simulink model "kiteModelNoAddedMassRapp"  (R2022a)
settings: Solver=VariableStepAuto  StartTime=0.0  StopTime=10.0  RelTol=1e-3
values from neighbouring files (symbols this model uses):
  aileronCmd = 0    [kiteModelNoAddedMassRapp_ts.m]
  alphaaI = 5    [kiteModelNoAddedMassRapp_ts.m]
  azI = 0    [kiteModelNoAddedMassRapp_ts.m]
  betaaI = 5    [kiteModelNoAddedMassRapp_ts.m]
  elevatorCmd = 4    [kiteModelNoAddedMassRapp_ts.m]
  elI = 20    [kiteModelNoAddedMassRapp_ts.m]
  htI = 100    [kiteModelNoAddedMassRapp_ts.m]
  J = vhcl.inertia_CM.Value    [kiteModelNoAddedMassRapp_ts.m]
  Jinv = inv(J)    [kiteModelNoAddedMassRapp_ts.m]
  m = vhcl.mass.Value    [kiteModelNoAddedMassRapp_ts.m]
  pbI = 0    [kiteModelNoAddedMassRapp_ts.m]
  phitI = 0    [kiteModelNoAddedMassRapp_ts.m]
  psitI = 0    [kiteModelNoAddedMassRapp_ts.m]
  qbI = 0    [kiteModelNoAddedMassRapp_ts.m]
  rbI = 0    [kiteModelNoAddedMassRapp_ts.m]
  rudderCmd = 0    [kiteModelNoAddedMassRapp_ts.m]
  thetatI = 0    [kiteModelNoAddedMassRapp_ts.m]
  vaI = 5    [kiteModelNoAddedMassRapp_ts.m]
  vW = 1    [kiteModelNoAddedMassRapp_ts.m]
undefined symbols (not defined in the file or in its folder): Copy_of_fluidDynamicSurface_cl, fluidDynamicSurface, fThrTanZConstant, vhcl
libraries: vrlib x12, dynamicPressure_ul x4, Copy_of_clAndCdCalculator_cl x4, alphaBetaLE_ul x4, localApparentWind_ul x4, rotateAboutVec x4, matrix_library x1
settings Model: Creator=jcreed2  LastModifiedBy=jcreed2
settings DebuggingCC: AlgebraicLoopMsg=none  ArtificialAlgebraicLoopMsg=none

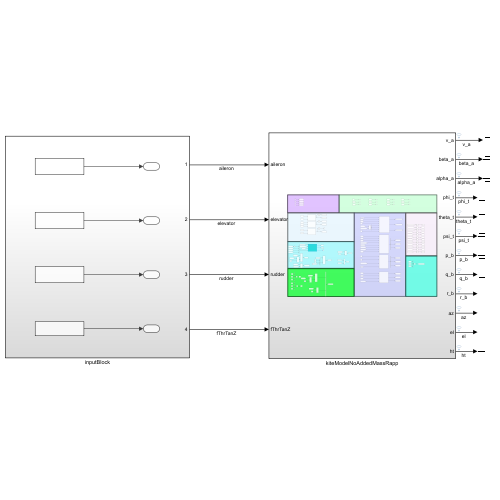
[thumbnail: Simulink's stored preview of the top-level diagram]
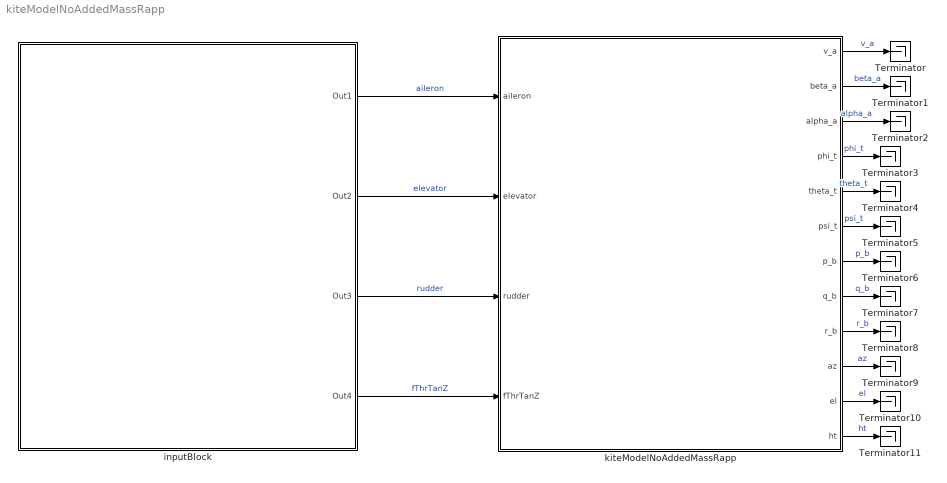
== system kiteModelNoAddedMassRapp ==
  Terminator{,1..11} (12 alike) : Terminator
  inputBlock : Subsystem
  kiteModelNoAddedMassRapp : Subsystem
  wires:
  kiteModelNoAddedMassRapp/1(v_a) -> Terminator/1  "v_a"
  kiteModelNoAddedMassRapp/2(beta_a) -> Terminator1/1  "beta_a"
  kiteModelNoAddedMassRapp/3(alpha_a) -> Terminator2/1  "alpha_a"
  kiteModelNoAddedMassRapp/4(phi_t) -> Terminator3/1  "phi_t"
  kiteModelNoAddedMassRapp/5(theta_t) -> Terminator4/1  "theta_t"
  kiteModelNoAddedMassRapp/6(psi_t) -> Terminator5/1  "psi_t"
  kiteModelNoAddedMassRapp/7(p_b) -> Terminator6/1  "p_b"
  kiteModelNoAddedMassRapp/8(q_b) -> Terminator7/1  "q_b"
  kiteModelNoAddedMassRapp/9(r_b) -> Terminator8/1  "r_b"
  kiteModelNoAddedMassRapp/10(az) -> Terminator9/1  "az"
  kiteModelNoAddedMassRapp/11(el) -> Terminator10/1  "el"
  kiteModelNoAddedMassRapp/12(ht) -> Terminator11/1  "ht"
  inputBlock/1(Out1) -> kiteModelNoAddedMassRapp/1(aileron)  "aileron"
  inputBlock/2(Out2) -> kiteModelNoAddedMassRapp/2(elevator)  "elevator"
  inputBlock/3(Out3) -> kiteModelNoAddedMassRapp/3(rudder)  "rudder"
  inputBlock/4(Out4) -> kiteModelNoAddedMassRapp/4(fThrTanZ)  "fThrTanZ"

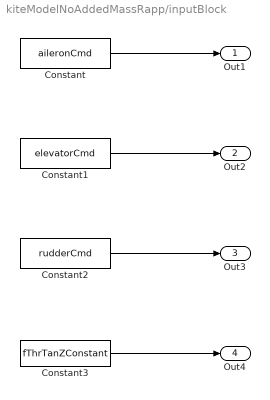
== system kiteModelNoAddedMassRapp/inputBlock ==
  Constant : Constant  Value=aileronCmd
  Constant1 : Constant  Value=elevatorCmd
  Constant2 : Constant  Value=rudderCmd
  Constant3 : Constant  Value=fThrTanZConstant
  Out1 : Outport
  Out2 : Outport  Port=2
  Out3 : Outport  Port=3
  Out4 : Outport  Port=4
  wires:
  Constant3/1 -> Out4/1
  Constant2/1 -> Out3/1
  Constant1/1 -> Out2/1
  Constant/1 -> Out1/1

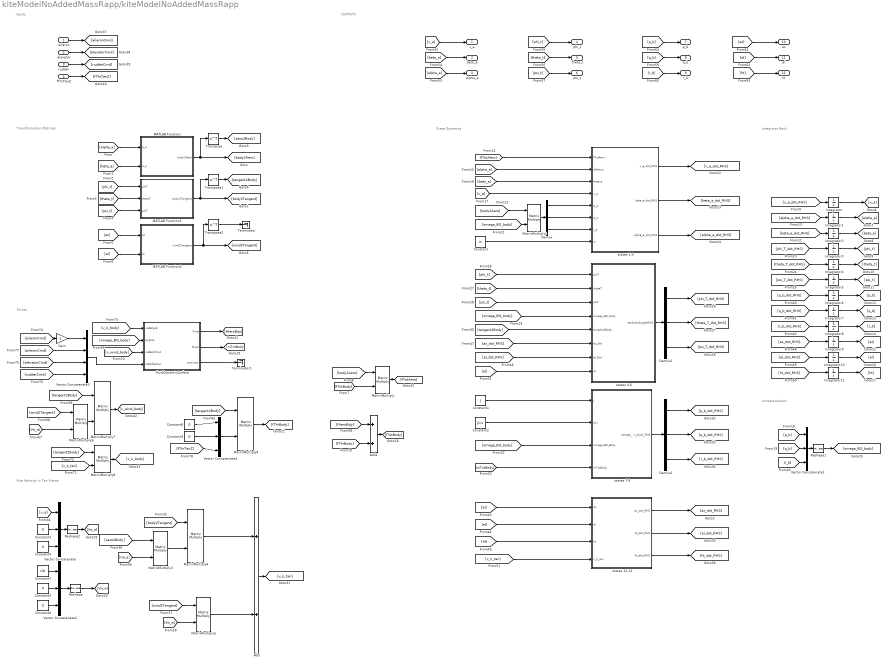
== system kiteModelNoAddedMassRapp/kiteModelNoAddedMassRapp ==
  note: OUTPUTS
  note: Inputs
  note: Kite Velocity in Tan Frame
  note: concatenations
  note: State Dynamics
  note: Forces
  note: Integrator Bank
  note: Transformation Matrices
  aileron : Inport
  elevator : Inport  Port=2
  rudder : Inport  Port=3
  fThrTanZ : Inport  Port=4
  Add : Sum
  Add1 : Sum
  Constant : Constant  Value=m
  Constant1 : Constant  Value=J
  Constant2 : Constant  Value=Jinv
  Constant{3..6,8..9} (6 alike) : Constant  Value=0
  Constant7 : Constant  Value=vW
  Demux : Demux  Outputs=3
  Demux1 : Demux  Outputs=3
  Demux2 : Demux  Outputs=3
  Gain : Gain  Gain=-1
  Integrator : Integrator  InitialCondition=vaI
  Integrator1 : Integrator  InitialCondition=alphaaI
  Integrator10 : Integrator  InitialCondition=elI
  Integrator11 : Integrator  InitialCondition=htI
  Integrator2 : Integrator  InitialCondition=betaaI
  Integrator3 : Integrator  InitialCondition=phitI
  Integrator4 : Integrator  InitialCondition=thetatI
  Integrator5 : Integrator  InitialCondition=psitI
  Integrator6 : Integrator  InitialCondition=pbI
  Integrator7 : Integrator  InitialCondition=qbI
  Integrator8 : Integrator  InitialCondition=rbI
  Integrator9 : Integrator  InitialCondition=azI
  MATLAB Function : MATLAB Function  TreatAsAtomicUnit=on
  MATLAB Function1 : MATLAB Function  TreatAsAtomicUnit=on
  MATLAB Function2 : MATLAB Function  TreatAsAtomicUnit=on
  MatrixMultiply{,2..9} (9 alike) : Product  Multiplication=Matrix(*)
  Reshape : Reshape  OutputDimensionality=Column vector (2-D)
  Reshape1 : Reshape  OutputDimensionality=Column vector (2-D)
  Reshape2 : Reshape  OutputDimensionality=Column vector (2-D)
  Terminator : Terminator
  Terminator1 : Terminator
  Transpose : Math  Operator=transpose
  Transpose1 : Math  Operator=transpose
  Transpose2 : Math  Operator=transpose
  Vector Concatenate{,1..2,4} (4 alike) : Concatenate  NumInputs=3
  Vector Concatenate3 : Concatenate  NumInputs=4
  fluidDynamicSurface : Subsystem  AncestorBlock=Copy_of_fluidDynamicSurface_cl/fluidDynamicSurface  mask{vcl=vhcl, fluidDensity=1000, fluidMomentArms=vhcl.fluidMomentArms.Value, fluidRefArea=vhcl.fluidRefArea.Value, wingTips=vhcl.wingTipPositions.Value}
      mask prompts: vcl "Vehicle object"; fluidDensity "Fluid density"; fluidMomentArms "Fluid Moment Arms"; fluidRefArea "Fluid Reference Area"; wingTips "Wing Tips"
      mask help:
      | Input must be an 1×N struct array with fields:
      |     refArea
      |     aeroCentPosVec
      |     spanUnitVec
      |     chordUnitVec
      |     CL
      |     CD
      |     alpha
      |     GainCL
      |     GainCD
      |
      | where N is the number of aerodynamic surfaces
      settings: MinAlgLoopOccurrences=on
  states 1-3 : Subsystem
  states 10-12 : Subsystem
  states 4-6 : Subsystem
  states 7-9 : Subsystem
  v_a : Outport
  beta_a : Outport  Port=2
  alpha_a : Outport  Port=3
  phi_t : Outport  Port=4
  theta_t : Outport  Port=5
  psi_t : Outport  Port=6
  p_b : Outport  Port=7
  q_b : Outport  Port=8
  r_b : Outport  Port=9
  az : Outport  Port=10
  el : Outport  Port=11
  ht : Outport  Port=12
  wires:
  Constant1/1 -> states 7-9/1(J)
  Constant2/1 -> states 7-9/2(Jinv)
  Demux/3 -> states 1-3/7(r_a)
  [omega_BO_body] -> states 7-9/3(omega_BO_Body)
  MatrixMultiply5/1 -> Add/2
  [tangent2Body] -> states 4-6/5(tangent2Body)
  [body2Aero] -> MatrixMultiply/1
  Integrator3/1 -> [phi_t]
  [phi_T_dot_RHS] -> Integrator3/1
  [body2Aero] -> MatrixMultiply2/1
  Integrator/1 -> [v_a]
  [el] -> states 4-6/8(el)
  Demux1/3 -> [psi_T_dot_RHS]
  states 1-3/2(beta_a_dot_RHS) -> [beta_a_dot_RHS]
  Constant6/1 -> Vector Concatenate2/3
  [psi_t] -> MATLAB Function1/3(psiT)
  Integrator1/1 -> [alpha_a]
  Vector Concatenate2/1 -> Reshape/1
  Transpose1/1 -> [tangent2Body]
  [Vw_w] -> MatrixMultiply5/2
  states 1-3/3(alpha_a_dot_RHS) -> [alpha_a_dot_RHS]
  Integrator5/1 -> [psi_t]
  [v_a] -> states 1-3/4(v_a)
  Integrator8/1 -> [r_b]
  Transpose/1 -> [aero2Body]
  Integrator4/1 -> [theta_t]
  [alpha_a] -> MATLAB Function/1(a_a)
  [alpha_a_dot_RHS] -> Integrator1/1
  [omega_BO_body] -> MatrixMultiply2/2
  states 10-12/3(ht_dot_RHS) -> [ht_dot_RHS]
  [r_b] -> Vector Concatenate1/3
  MatrixMultiply4/1 -> Add/1
  [theta_T_dot_RHS] -> Integrator4/1
  Integrator11/1 -> [ht]
  Demux/1 -> states 1-3/5(p_a)
  [beta_a_dot_RHS] -> Integrator2/1
  [p_b_dot_RHS] -> Integrator6/1
  [beta_a] -> MATLAB Function/2(b_a)
  Constant5/1 -> Vector Concatenate2/2
  [az] -> states 10-12/1(az)
  MATLAB Function/1(body2Aero) -> Transpose/1, [body2Aero]
  [v_a] -> Vector Concatenate/1
  Integrator6/1 -> [p_b]
  [v_k_tan] -> states 10-12/4(v_k_tan)
  [q_b_dot_RHS] -> Integrator7/1
  [phi_t] -> states 4-6/1(phiT)
  MatrixMultiply/1 -> [fTotAero]
  Integrator2/1 -> [beta_a]
  MatrixMultiply2/1 -> Demux/1
  Demux2/3 -> [r_b_dot_RHS]
  Integrator7/1 -> [q_b]
  states 7-9/1(omega_BO_Dot_body_RHS) -> Demux2/1
  Integrator10/1 -> [el]
  Reshape1/1 -> [omega_BO_body]
  [fTotBody] -> MatrixMultiply/2
  [el] -> MATLAB Function2/2(el)
  Constant3/1 -> Vector Concatenate/2
  MATLAB Function1/1(body2Tangent) -> Transpose1/1, [body2Tangent]
  [psi_t] -> states 4-6/3(psiT)
  MATLAB Function2/1(wind2Tangent) -> Transpose2/1, [wind2Tangent]
  [p_b] -> Vector Concatenate1/1
  [phi_t] -> MATLAB Function1/1(phiT)
  [q_b] -> Vector Concatenate1/2
  Integrator9/1 -> [az]
  [az_dot_RHS] -> Integrator9/1
  [ht_dot_RHS] -> Integrator11/1
  [az] -> MATLAB Function2/1(az)
  [theta_t] -> MATLAB Function1/2(thetaT)
  [r_b_dot_RHS] -> Integrator8/1
  [el_dot_RHS] -> Integrator10/1
  [mTotBody] -> states 7-9/4(mTotBody)
  [theta_t] -> states 4-6/2(thetaT)
  Constant7/1 -> Vector Concatenate2/1
  Demux/2 -> states 1-3/6(q_a)
  Vector Concatenate/1 -> Reshape2/1
  Transpose2/1 -> Terminator/1
  [fTotAero] -> states 1-3/1(fTotAero)
  [beta_a] -> states 1-3/3(beta_a)
  Demux1/2 -> [theta_T_dot_RHS]
  Demux1/1 -> [phi_T_dot_RHS]
  [body2Tangent] -> MatrixMultiply4/1
  [alpha_a] -> states 1-3/2(alpha_a)
  Demux2/2 -> [q_b_dot_RHS]
  [aero2Body] -> MatrixMultiply3/1
  [el_dot_RHS] -> states 4-6/7(el_Dot)
  Constant4/1 -> Vector Concatenate/3
  [psi_T_dot_RHS] -> Integrator5/1
  Constant/1 -> states 1-3/8(m)
  [el] -> states 10-12/2(el)
  [v_a_dot_RHS] -> Integrator/1
  states 1-3/1(v_a_dot_RHS) -> [v_a_dot_RHS]
  [ht] -> states 10-12/3(ht)
  MatrixMultiply3/1 -> MatrixMultiply4/2
  Demux2/1 -> [p_b_dot_RHS]
  states 10-12/1(az_dot_RHS) -> [az_dot_RHS]
  Vector Concatenate1/1 -> Reshape1/1
  states 10-12/2(el_dot_RHS) -> [el_dot_RHS]
  [Va_a] -> MatrixMultiply3/2
  Add/1 -> [v_k_tan]
  states 4-6/1(tanEulerAnglesRHS) -> Demux1/1
  [omega_BO_body] -> states 4-6/4(omega_BO_body)
  [wind2Tangent] -> MatrixMultiply5/1
  [az_dot_RHS] -> states 4-6/6(az_dot)
  Add1/1 -> [fTotBody]
  aileron/1 -> [aileronCmd]
  elevator/1 -> [elevatorCmd]
  rudder/1 -> [rudderCmd]
  fThrTanZ/1 -> [fThrTanZ]
  [alpha_a] -> alpha_a/1
  [beta_a] -> beta_a/1
  [v_a] -> v_a/1
  [phi_t] -> phi_t/1
  [theta_t] -> theta_t/1
  [psi_t] -> psi_t/1
  [p_b] -> p_b/1
  [q_b] -> q_b/1
  [r_b] -> r_b/1
  [az] -> az/1
  [el] -> el/1
  [ht] -> ht/1
  fluidDynamicSurface/3(powLoss) -> Terminator1/1
  fluidDynamicSurface/2(Mnet) -> [mTotBody]
  fluidDynamicSurface/1(Fnet) -> [fAeroBdy]
  [fAeroBdy] -> Add1/1
  [fThrBody] -> Add1/2
  [omega_BO_body] -> fluidDynamicSurface/2(angVel)
  [Vw_w] -> MatrixMultiply6/2
  [wind2Tangent] -> MatrixMultiply6/1
  MatrixMultiply6/1 -> MatrixMultiply7/2
  [tangent2Body] -> MatrixMultiply7/1
  MatrixMultiply7/1 -> [v_wind_body]
  [v_wind_body] -> fluidDynamicSurface/3(velBdyWind)
  [tangent2Body] -> MatrixMultiply8/1
  [v_k_tan] -> MatrixMultiply8/2
  MatrixMultiply8/1 -> [v_k_body]
  [v_k_body] -> fluidDynamicSurface/1(velBdyLE)
  Vector Concatenate3/1 -> fluidDynamicSurface/4(csDeflection)
  Gain/1 -> Vector Concatenate3/1
  [aileronCmd] -> Gain/1
  [elevatorCmd] -> Vector Concatenate3/3
  [rudderCmd] -> Vector Concatenate3/4
  [aileronCmd] -> Vector Concatenate3/2
  Reshape/1 -> [Vw_w]
  Reshape2/1 -> [Va_a]
  [fThrTanZ] -> Vector Concatenate4/3
  MatrixMultiply9/1 -> [fThrBody]
  [tangent2Body] -> MatrixMultiply9/1
  Vector Concatenate4/1 -> MatrixMultiply9/2
  Constant8/1 -> Vector Concatenate4/1
  Constant9/1 -> Vector Concatenate4/2

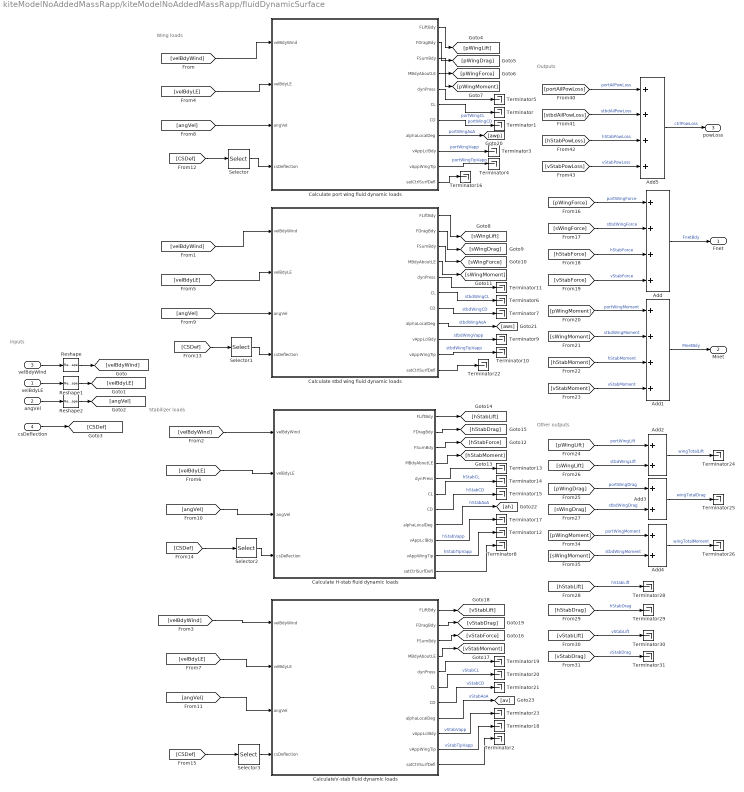
== system kiteModelNoAddedMassRapp/kiteModelNoAddedMassRapp/fluidDynamicSurface ==
  note: inputs
  note: Stabilizer loads
  note: WIng loads
  note: Outputs
  note: Other outputs
  velBdyLE : Inport
  angVel : Inport  Port=2
  velBdyWind : Inport  Port=3
  csDeflection : Inport  Port=4
  Add : Sum  Inputs=++++
  Add1 : Sum  Inputs=++++
  Add2 : Sum
  Add3 : Sum
  Add4 : Sum
  Add5 : Sum  Inputs=++++
  Calculate H-stab fluid dynamic loads : Subsystem  AncestorBlock=calcFluidDynamicLoads/Calculate fluid dynamic loads  mask{aSurf=vhcl.hStab, sRef=fluidRefArea, rArm_LE=fluidMomentArms(:,3), rTip_LE=wingTips(:,3), fluidDensity=fluidDensity}
      mask prompts: aSurf "Aerosurf object"; sRef "Reference area"; rArm_LE "Moment arm wrt wing LE"; rTip_LE "Surface tip wrt wing LE"; fluidDensity "Fluid density"
  Calculate port wing fluid dynamic loads : Subsystem  AncestorBlock=calcFluidDynamicLoads/Calculate fluid dynamic loads  mask{aSurf=vhcl.portWing, sRef=fluidRefArea, rArm_LE=fluidMomentArms(:,1), rTip_LE=wingTips(:,1), fluidDensity=fluidDensity}
      mask prompts: aSurf "Aerosurf object"; sRef "Reference area"; rArm_LE "Moment arm wrt wing LE"; rTip_LE "Surface tip wrt wing LE"; fluidDensity "Fluid density"
  Calculate stbd wing fluid dynamic loads : Subsystem  AncestorBlock=calcFluidDynamicLoads/Calculate fluid dynamic loads  mask{aSurf=vhcl.stbdWing, sRef=fluidRefArea, rArm_LE=fluidMomentArms(:,2), rTip_LE=wingTips(:,2), fluidDensity=fluidDensity}
      mask prompts: aSurf "Aerosurf object"; sRef "Reference area"; rArm_LE "Moment arm wrt wing LE"; rTip_LE "Surface tip wrt wing LE"; fluidDensity "Fluid density"
  CalculateV-stab fluid dynamic loads : Subsystem  AncestorBlock=calcFluidDynamicLoads/Calculate fluid dynamic loads  mask{aSurf=vhcl.vStab, sRef=fluidRefArea, rArm_LE=fluidMomentArms(:,4), rTip_LE=wingTips(:,4), fluidDensity=fluidDensity}
      mask prompts: aSurf "Aerosurf object"; sRef "Reference area"; rArm_LE "Moment arm wrt wing LE"; rTip_LE "Surface tip wrt wing LE"; fluidDensity "Fluid density"
  Reshape : Reshape  OutputDimensionality=Column vector (2-D)
  Reshape1 : Reshape  OutputDimensionality=Column vector (2-D)
  Reshape2 : Reshape  OutputDimensionality=Column vector (2-D)
  Selector : Selector  InputPortWidth=4  IndexOptions=Index vector (dialog)  Indices=1  OutputSizes=1
  Selector1 : Selector  InputPortWidth=4  IndexOptions=Index vector (dialog)  Indices=2  OutputSizes=1
  Selector2 : Selector  InputPortWidth=4  IndexOptions=Index vector (dialog)  Indices=3  OutputSizes=1
  Selector3 : Selector  InputPortWidth=4  IndexOptions=Index vector (dialog)  Indices=4  OutputSizes=1
  Terminator{,1..26,28..31} (31 alike) : Terminator
  Fnet : Outport
  Mnet : Outport  Port=2
  powLoss : Outport  Port=3
  wires:
  [vStabPowLoss] -> Add5/4  "vStabPowLoss"
  [hStabPowLoss] -> Add5/3  "hStabPowLoss"
  Add5/1 -> powLoss/1  "ctrlPowLoss"
  [stbdAilPowLoss] -> Add5/2  "stbdAilPowLoss"
  [portAilPowLoss] -> Add5/1  "portAilPowLoss"
  CalculateV-stab fluid dynamic loads/11(satCtrlSurfDefl) -> Terminator2/1
  Calculate H-stab fluid dynamic loads/11(satCtrlSurfDefl) -> Terminator8/1
  Calculate stbd wing fluid dynamic loads/11(satCtrlSurfDefl) -> Terminator22/1
  Calculate port wing fluid dynamic loads/11(satCtrlSurfDefl) -> Terminator16/1
  [sWingMoment] -> Add4/2  "stbdWingMoment"
  [pWingMoment] -> Add4/1  "portWingMoment"
  Add4/1 -> Terminator26/1  "wingTotalMoment"
  Add3/1 -> Terminator25/1  "wingTotalDrag"
  Add2/1 -> Terminator24/1  "wingTotalLift"
  [velBdyWind] -> CalculateV-stab fluid dynamic loads/1(velBdyWind)
  [velBdyWind] -> Calculate H-stab fluid dynamic loads/1(velBdyWind)
  [velBdyWind] -> Calculate stbd wing fluid dynamic loads/1(velBdyWind)
  [velBdyWind] -> Calculate port wing fluid dynamic loads/1(velBdyWind)
  [pWingLift] -> Add2/1  "portWingLift"
  [pWingDrag] -> Add3/1  "portWingDrag"
  [sWingLift] -> Add2/2  "stbdWingLift"
  [sWingDrag] -> Add3/2  "stbdWingDrag"
  [hStabLift] -> Terminator28/1  "hStabLift"
  [hStabDrag] -> Terminator29/1  "hStabDrag"
  [vStabLift] -> Terminator30/1  "vStabLift"
  [vStabDrag] -> Terminator31/1  "vStabDrag"
  [pWingMoment] -> Add1/1  "portWingMoment"
  [sWingMoment] -> Add1/2  "stbdWingMoment"
  [hStabMoment] -> Add1/3  "hStabMoment"
  [vStabMoment] -> Add1/4  "vStabMoment"
  Add1/1 -> Mnet/1  "MnetBdy"
  Add/1 -> Fnet/1  "FnetBdy"
  [hStabForce] -> Add/3  "hStabForce"
  [vStabForce] -> Add/4  "vStabForce"
  [sWingForce] -> Add/2  "stbdWingForce"
  [pWingForce] -> Add/1  "portWingForce"
  CalculateV-stab fluid dynamic loads/7(CD) -> Terminator21/1  "vStabCD"
  CalculateV-stab fluid dynamic loads/10(vAppWingTip) -> Terminator18/1  "vStabTipVapp"
  CalculateV-stab fluid dynamic loads/2(FDragBdy) -> [vStabDrag]
  CalculateV-stab fluid dynamic loads/5(dynPress) -> Terminator19/1
  CalculateV-stab fluid dynamic loads/8(alphaLocalDeg) -> [av]  "vStabAoA"
  CalculateV-stab fluid dynamic loads/4(MBdyAboutLE) -> [vStabMoment]
  CalculateV-stab fluid dynamic loads/9(vAppLclBdy) -> Terminator23/1  "vStabVapp"
  CalculateV-stab fluid dynamic loads/6(CL) -> Terminator20/1  "vStabCL"
  CalculateV-stab fluid dynamic loads/1(FLiftBdy) -> [vStabLift]
  CalculateV-stab fluid dynamic loads/3(FSumBdy) -> [vStabForce]
  Calculate H-stab fluid dynamic loads/9(vAppLclBdy) -> Terminator17/1  "hStabVapp"
  Calculate H-stab fluid dynamic loads/10(vAppWingTip) -> Terminator12/1  "hStabTipVapp"
  Calculate H-stab fluid dynamic loads/8(alphaLocalDeg) -> [ah]  "hStabAoA"
  Calculate H-stab fluid dynamic loads/3(FSumBdy) -> [hStabForce]
  Calculate H-stab fluid dynamic loads/6(CL) -> Terminator14/1  "hStabCL"
  Calculate H-stab fluid dynamic loads/1(FLiftBdy) -> [hStabLift]
  Calculate H-stab fluid dynamic loads/7(CD) -> Terminator15/1  "hStabCD"
  Calculate H-stab fluid dynamic loads/5(dynPress) -> Terminator13/1
  Calculate H-stab fluid dynamic loads/4(MBdyAboutLE) -> [hStabMoment]
  Calculate H-stab fluid dynamic loads/2(FDragBdy) -> [hStabDrag]
  Calculate stbd wing fluid dynamic loads/4(MBdyAboutLE) -> [sWingMoment]
  Calculate stbd wing fluid dynamic loads/3(FSumBdy) -> [sWingForce]
  Calculate stbd wing fluid dynamic loads/2(FDragBdy) -> [sWingDrag]
  Calculate stbd wing fluid dynamic loads/1(FLiftBdy) -> [sWingLift]
  Calculate stbd wing fluid dynamic loads/10(vAppWingTip) -> Terminator10/1  "stbdWingTipVapp"
  Calculate stbd wing fluid dynamic loads/7(CD) -> Terminator7/1  "stbdWingCD"
  Calculate stbd wing fluid dynamic loads/8(alphaLocalDeg) -> [aws]  "stbdWingAoA"
  Calculate stbd wing fluid dynamic loads/6(CL) -> Terminator6/1  "stbdWingCL"
  Calculate stbd wing fluid dynamic loads/9(vAppLclBdy) -> Terminator9/1  "stbdWingVapp"
  Calculate stbd wing fluid dynamic loads/5(dynPress) -> Terminator11/1
  Calculate port wing fluid dynamic loads/5(dynPress) -> Terminator5/1
  Calculate port wing fluid dynamic loads/10(vAppWingTip) -> Terminator4/1  "portWingTipVapp"
  Calculate port wing fluid dynamic loads/9(vAppLclBdy) -> Terminator3/1  "portWingVapp"
  Calculate port wing fluid dynamic loads/8(alphaLocalDeg) -> [awp]  "portWingAoA"
  Calculate port wing fluid dynamic loads/7(CD) -> Terminator1/1  "portWingCD"
  Calculate port wing fluid dynamic loads/6(CL) -> Terminator/1  "portWingCL"
  Calculate port wing fluid dynamic loads/4(MBdyAboutLE) -> [pWingMoment]
  Calculate port wing fluid dynamic loads/3(FSumBdy) -> [pWingForce]
  Calculate port wing fluid dynamic loads/2(FDragBdy) -> [pWingDrag]
  Calculate port wing fluid dynamic loads/1(FLiftBdy) -> [pWingLift]
  Selector3/1 -> CalculateV-stab fluid dynamic loads/4(csDeflection)
  Selector2/1 -> Calculate H-stab fluid dynamic loads/4(csDeflection)
  [CSDef] -> Selector3/1
  [CSDef] -> Selector2/1
  [CSDef] -> Selector1/1
  Selector1/1 -> Calculate stbd wing fluid dynamic loads/4(csDeflection)
  Selector/1 -> Calculate port wing fluid dynamic loads/4(csDeflection)
  [CSDef] -> Selector/1
  [angVel] -> CalculateV-stab fluid dynamic loads/3(angVel)
  [angVel] -> Calculate H-stab fluid dynamic loads/3(angVel)
  [angVel] -> Calculate stbd wing fluid dynamic loads/3(angVel)
  [angVel] -> Calculate port wing fluid dynamic loads/3(angVel)
  [velBdyLE] -> CalculateV-stab fluid dynamic loads/2(velBdyLE)
  [velBdyLE] -> Calculate H-stab fluid dynamic loads/2(velBdyLE)
  [velBdyLE] -> Calculate stbd wing fluid dynamic loads/2(velBdyLE)
  [velBdyLE] -> Calculate port wing fluid dynamic loads/2(velBdyLE)
  csDeflection/1 -> [CSDef]
  velBdyWind/1 -> Reshape/1
  velBdyLE/1 -> Reshape1/1
  angVel/1 -> Reshape2/1
  Reshape/1 -> [velBdyWind]
  Reshape1/1 -> [velBdyLE]
  Reshape2/1 -> [angVel]

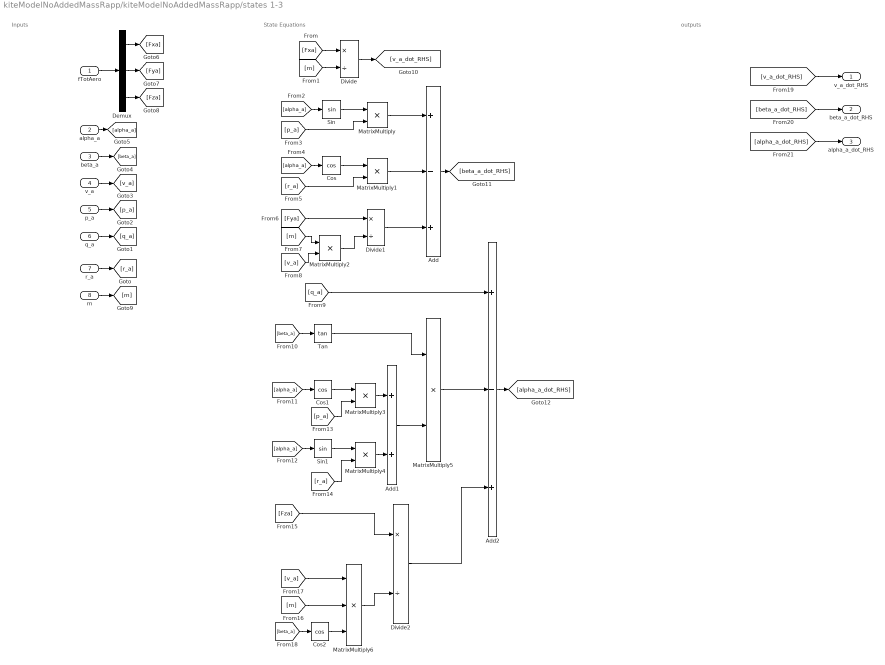
== system kiteModelNoAddedMassRapp/kiteModelNoAddedMassRapp/states 1-3 ==
  note: State Equations
  note: Inputs
  note: outputs
  fTotAero : Inport
  alpha_a : Inport  Port=2
  beta_a : Inport  Port=3
  v_a : Inport  Port=4
  p_a : Inport  Port=5
  q_a : Inport  Port=6
  r_a : Inport  Port=7
  m : Inport  Port=8
  Add : Sum  Inputs=+-+
  Add1 : Sum
  Add2 : Sum  Inputs=+-+
  Cos : Trigonometry  Operator=cos
  Cos1 : Trigonometry  Operator=cos
  Cos2 : Trigonometry  Operator=cos
  Demux : Demux  Outputs=3
  Divide : Product  Inputs=*/
  Divide1 : Product  Inputs=*/
  Divide2 : Product  Inputs=*/
  MatrixMultiply{,1..5} (6 alike) : Product
  MatrixMultiply6 : Product  Inputs=3
  Sin : Trigonometry
  Sin1 : Trigonometry
  Tan : Trigonometry  Operator=tan
  v_a_dot_RHS : Outport
  beta_a_dot_RHS : Outport  Port=2
  alpha_a_dot_RHS : Outport  Port=3
  wires:
  r_a/1 -> [r_a]
  q_a/1 -> [q_a]
  p_a/1 -> [p_a]
  v_a/1 -> [v_a]
  beta_a/1 -> [beta_a]
  alpha_a/1 -> [alpha_a]
  fTotAero/1 -> Demux/1
  Demux/1 -> [Fxa]
  Demux/2 -> [Fya]
  Demux/3 -> [Fza]
  m/1 -> [m]
  [Fxa] -> Divide/1
  [m] -> Divide/2
  Divide/1 -> [v_a_dot_RHS]
  [alpha_a] -> Sin/1
  Sin/1 -> MatrixMultiply/1
  [p_a] -> MatrixMultiply/2
  [alpha_a] -> Cos/1
  Cos/1 -> MatrixMultiply1/1
  [r_a] -> MatrixMultiply1/2
  [Fya] -> Divide1/1
  [m] -> MatrixMultiply2/1
  [v_a] -> MatrixMultiply2/2
  MatrixMultiply2/1 -> Divide1/2
  MatrixMultiply/1 -> Add/1
  MatrixMultiply1/1 -> Add/2
  Divide1/1 -> Add/3
  Add/1 -> [beta_a_dot_RHS]
  [beta_a] -> Tan/1
  [alpha_a] -> Cos1/1
  [alpha_a] -> Sin1/1
  Cos1/1 -> MatrixMultiply3/1
  Sin1/1 -> MatrixMultiply4/1
  [p_a] -> MatrixMultiply3/2
  [r_a] -> MatrixMultiply4/2
  MatrixMultiply3/1 -> Add1/1
  MatrixMultiply4/1 -> Add1/2
  Add1/1 -> MatrixMultiply5/2
  Tan/1 -> MatrixMultiply5/1
  [Fza] -> Divide2/1
  MatrixMultiply6/1 -> Divide2/2
  [v_a] -> MatrixMultiply6/1
  [m] -> MatrixMultiply6/2
  Cos2/1 -> MatrixMultiply6/3
  [beta_a] -> Cos2/1
  Divide2/1 -> Add2/3
  MatrixMultiply5/1 -> Add2/2
  [q_a] -> Add2/1
  Add2/1 -> [alpha_a_dot_RHS]
  [v_a_dot_RHS] -> v_a_dot_RHS/1
  [beta_a_dot_RHS] -> beta_a_dot_RHS/1
  [alpha_a_dot_RHS] -> alpha_a_dot_RHS/1

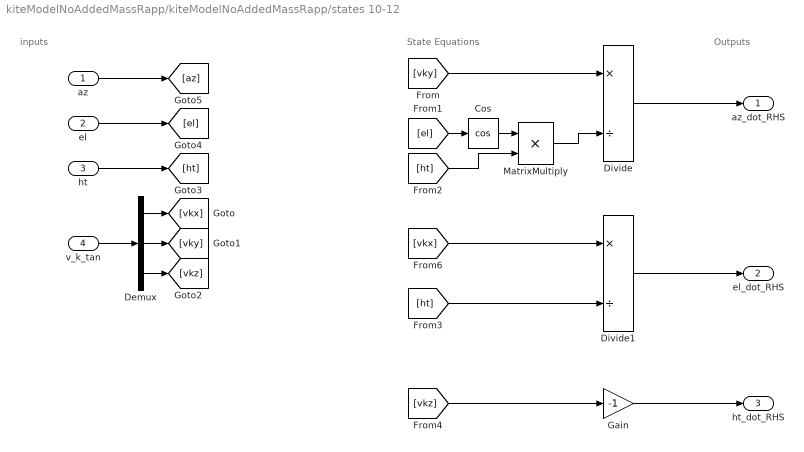
== system kiteModelNoAddedMassRapp/kiteModelNoAddedMassRapp/states 10-12 ==
  note: Outputs
  note: State Equations
  note: inputs
  az : Inport
  el : Inport  Port=2
  ht : Inport  Port=3
  v_k_tan : Inport  Port=4
  Cos : Trigonometry  Operator=cos
  Demux : Demux  Outputs=3
  Divide : Product  Inputs=*/
  Divide1 : Product  Inputs=*/
  Gain : Gain  Gain=-1
  MatrixMultiply : Product
  az_dot_RHS : Outport
  el_dot_RHS : Outport  Port=2
  ht_dot_RHS : Outport  Port=3
  wires:
  v_k_tan/1 -> Demux/1
  Demux/1 -> [vkx]
  Demux/2 -> [vky]
  Demux/3 -> [vkz]
  ht/1 -> [ht]
  el/1 -> [el]
  az/1 -> [az]
  [vky] -> Divide/1
  [el] -> Cos/1
  Cos/1 -> MatrixMultiply/1
  MatrixMultiply/1 -> Divide/2
  [ht] -> MatrixMultiply/2
  [vkx] -> Divide1/1
  [ht] -> Divide1/2
  [vkz] -> Gain/1
  Gain/1 -> ht_dot_RHS/1
  Divide1/1 -> el_dot_RHS/1
  Divide/1 -> az_dot_RHS/1

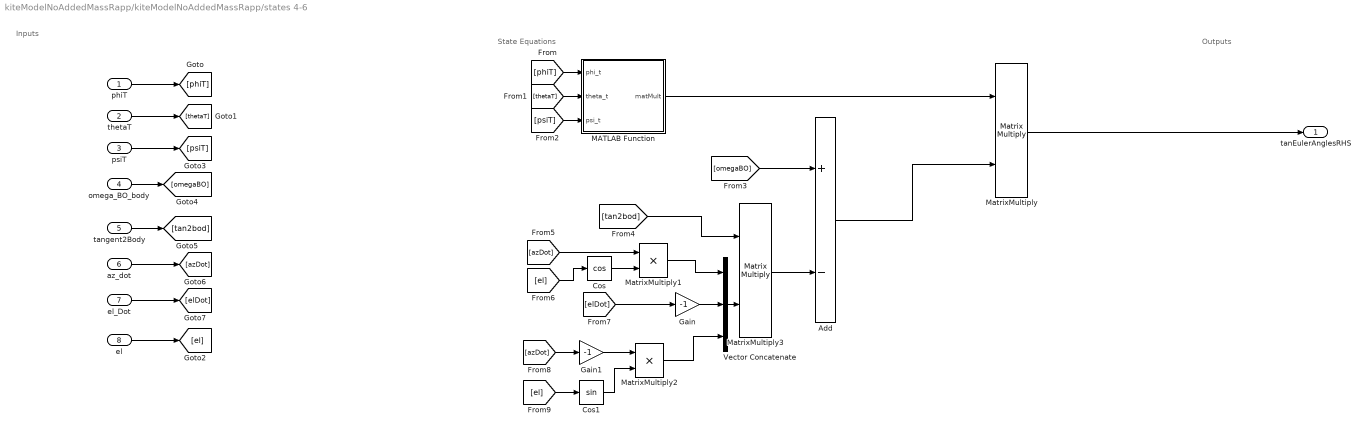
== system kiteModelNoAddedMassRapp/kiteModelNoAddedMassRapp/states 4-6 ==
  note: Outputs
  note: State Equations
  note: Inputs
  phiT : Inport
  thetaT : Inport  Port=2
  psiT : Inport  Port=3
  omega_BO_body : Inport  Port=4
  tangent2Body : Inport  Port=5
  az_dot : Inport  Port=6
  el_Dot : Inport  Port=7
  el : Inport  Port=8
  Add : Sum  Inputs=+-
  Cos : Trigonometry  Operator=cos
  Cos1 : Trigonometry
  Gain : Gain  Gain=-1
  Gain1 : Gain  Gain=-1
  MATLAB Function : MATLAB Function  TreatAsAtomicUnit=on
  MatrixMultiply : Product  Multiplication=Matrix(*)
  MatrixMultiply1 : Product
  MatrixMultiply2 : Product
  MatrixMultiply3 : Product  Multiplication=Matrix(*)
  Vector Concatenate : Concatenate  NumInputs=3
  tanEulerAnglesRHS : Outport
  wires:
  phiT/1 -> [phiT]
  thetaT/1 -> [thetaT]
  el_Dot/1 -> [elDot]
  az_dot/1 -> [azDot]
  tangent2Body/1 -> [tan2bod]
  omega_BO_body/1 -> [omegaBO]
  psiT/1 -> [psiT]
  [phiT] -> MATLAB Function/1(phi_t)
  [thetaT] -> MATLAB Function/2(theta_t)
  [psiT] -> MATLAB Function/3(psi_t)
  MATLAB Function/1(matMult) -> MatrixMultiply/1
  [omegaBO] -> Add/1
  [azDot] -> MatrixMultiply1/1
  el/1 -> [el]
  [el] -> Cos/1
  MatrixMultiply1/1 -> Vector Concatenate/1
  Cos/1 -> MatrixMultiply1/2
  Gain/1 -> Vector Concatenate/2
  [elDot] -> Gain/1
  MatrixMultiply2/1 -> Vector Concatenate/3
  [azDot] -> Gain1/1
  Gain1/1 -> MatrixMultiply2/1
  Cos1/1 -> MatrixMultiply2/2
  [el] -> Cos1/1
  Vector Concatenate/1 -> MatrixMultiply3/2
  [tan2bod] -> MatrixMultiply3/1
  MatrixMultiply3/1 -> Add/2
  Add/1 -> MatrixMultiply/2
  MatrixMultiply/1 -> tanEulerAnglesRHS/1

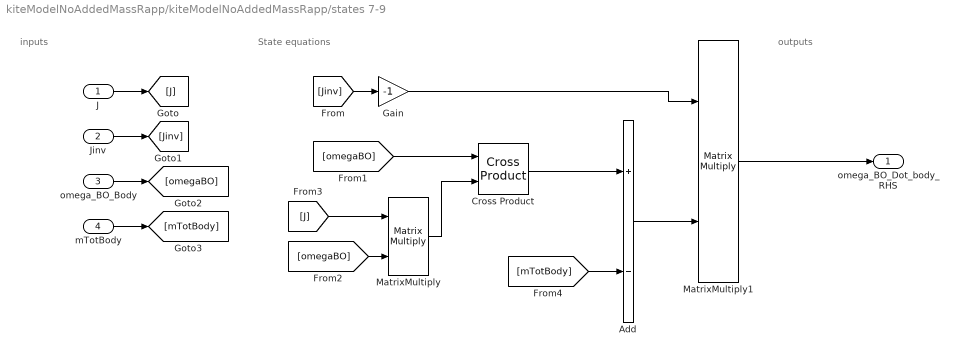
== system kiteModelNoAddedMassRapp/kiteModelNoAddedMassRapp/states 7-9 ==
  note: outputs
  note: State equations
  note: inputs
  J : Inport
  Jinv : Inport  Port=2
  omega_BO_Body : Inport  Port=3
  mTotBody : Inport  Port=4
  Add : Sum  Inputs=+-
  Cross Product : matrix_library/Cross Product
      settings: SourceProductBaseCode=SL
  Gain : Gain  Gain=-1
  MatrixMultiply : Product  Multiplication=Matrix(*)
  MatrixMultiply1 : Product  Multiplication=Matrix(*)
  omega_BO_Dot_body_RHS : Outport
  wires:
  J/1 -> [J]
  Jinv/1 -> [Jinv]
  omega_BO_Body/1 -> [omegaBO]
  mTotBody/1 -> [mTotBody]
  [Jinv] -> Gain/1
  [omegaBO] -> Cross Product/1
  MatrixMultiply/1 -> Cross Product/2
  [omegaBO] -> MatrixMultiply/2
  [J] -> MatrixMultiply/1
  [mTotBody] -> Add/2
  Cross Product/1 -> Add/1
  Gain/1 -> MatrixMultiply1/1
  Add/1 -> MatrixMultiply1/2
  MatrixMultiply1/1 -> omega_BO_Dot_body_RHS/1

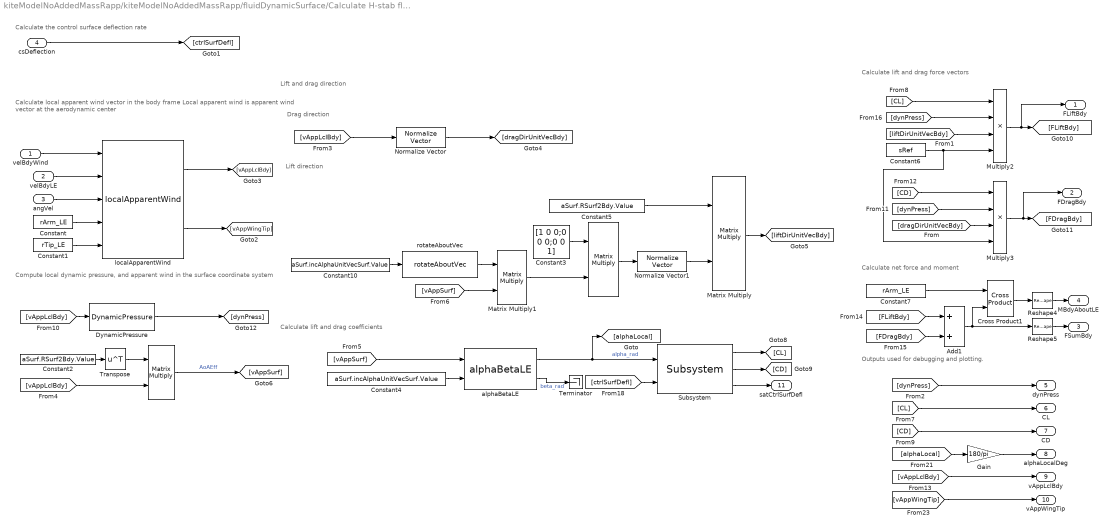
== system kiteModelNoAddedMassRapp/kiteModelNoAddedMassRapp/fluidDynamicSurface/Calculate H-stab fluid dynamic loads ==
  note: Calculate the control surface deflection rate
  note: Lift and drag direction
  note: Lift direction
  note: Drag direction
  note: Compute local dynamic pressure,
      | and apparent wind in the surface coordinate system
  note: Calculate local apparent wind vector in the body frame
      | Local apparent wind is apparent wind vector at the aerodynamic center
  note: Calculate lift and drag coefficients
  note: Calculate net force and moment
  note: Outputs used for debugging and plotting.
  note: Calculate lift and drag force vectors
  velBdyWind : Inport
  velBdyLE : Inport  Port=2
  angVel : Inport  Port=3
  csDeflection : Inport  Port=4
  " " : Product  Multiplication=Matrix(*)
  "  " : Product  Multiplication=Matrix(*)
  Add1 : Sum
  Constant : Constant  Value=rArm_LE  VectorParams1D=off
  Constant1 : Constant  Value=rTip_LE  VectorParams1D=off
  Constant10 : Constant  Value=aSurf.incAlphaUnitVecSurf.Value  VectorParams1D=off
  Constant2 : Constant  Value=aSurf.RSurf2Bdy.Value  VectorParams1D=off
  Constant3 : Constant  Value=[1 0 0;0 0 0;0 0 1]  VectorParams1D=off
  Constant4 : Constant  Value=aSurf.incAlphaUnitVecSurf.Value  VectorParams1D=off
  Constant5 : Constant  Value=aSurf.RSurf2Bdy.Value  VectorParams1D=off
  Constant6 : Constant  Value=sRef
  Constant7 : Constant  Value=rArm_LE  VectorParams1D=off
  Cross Product1 : vrlib/Utilities/Cross Product
  DynamicPressure : dynamicPressure_ul/DynamicPressure  rho=fluidDensity
  Gain : Gain  Gain=180/pi
  Matrix Multiply : Product  Multiplication=Matrix(*)
  Matrix Multiply1 : Product  Multiplication=Matrix(*)
  Multiply2 : Product  Inputs=4
  Multiply3 : Product  Inputs=4
  Normalize Vector : vrlib/Utilities/Normalize Vector  maxzero=0
  Normalize Vector1 : vrlib/Utilities/Normalize Vector  maxzero=0
  Reshape4 : Reshape  OutputDimensionality=Column vector (2-D)
  Reshape5 : Reshape  OutputDimensionality=Column vector (2-D)
  Subsystem : Copy_of_clAndCdCalculator_cl/Subsystem  aSurf=aSurf
  Terminator : Terminator
  Transpose : Math  Operator=transpose  SignedPower=on
  alphaBetaLE : alphaBetaLE_ul/alphaBetaLE  SystemSampleTime=-1  VariantActivationTime=update diagram  Latency=0  AutoFrameSizeCalculation=off
  localApparentWind : localApparentWind_ul/localApparentWind  SystemSampleTime=-1  VariantActivationTime=update diagram  Latency=0  AutoFrameSizeCalculation=off
  rotateAboutVec : rotateAboutVec/rotateAboutVec  ang=90
  FLiftBdy : Outport  VectorParamsAs1DForOutWhenUnconnected=off
  FDragBdy : Outport  Port=2  VectorParamsAs1DForOutWhenUnconnected=off
  FSumBdy : Outport  Port=3  VectorParamsAs1DForOutWhenUnconnected=off
  MBdyAboutLE : Outport  Port=4  PortDimensions=[3 1]  VectorParamsAs1DForOutWhenUnconnected=off
  dynPress : Outport  Port=5  VectorParamsAs1DForOutWhenUnconnected=off
  CL : Outport  Port=6  VectorParamsAs1DForOutWhenUnconnected=off
  CD : Outport  Port=7  VectorParamsAs1DForOutWhenUnconnected=off
  alphaLocalDeg : Outport  Port=8  VectorParamsAs1DForOutWhenUnconnected=off
  vAppLclBdy : Outport  Port=9  VectorParamsAs1DForOutWhenUnconnected=off
  vAppWingTip : Outport  Port=10  VectorParamsAs1DForOutWhenUnconnected=off
  satCtrlSurfDefl : Outport  Port=11
  wires:
  velBdyLE/1 -> localApparentWind/2
  angVel/1 -> localApparentWind/3
  Constant/1 -> localApparentWind/4
  Constant1/1 -> localApparentWind/5
  Constant2/1 -> Transpose/1
  Transpose/1 -> "  "/1
  Constant3/1 -> " "/1
  rotateAboutVec/1 -> Matrix Multiply1/1
  Matrix Multiply/1 -> [liftDirUnitVecBdy]
  Normalize Vector1/1 -> Matrix Multiply/2
  Constant10/1 -> rotateAboutVec/1
  Matrix Multiply1/1 -> " "/2
  " "/1 -> Normalize Vector1/1
  Constant5/1 -> Matrix Multiply/1
  [vAppSurf] -> Matrix Multiply1/2
  Normalize Vector/1 -> [dragDirUnitVecBdy]
  [vAppLclBdy] -> Normalize Vector/1
  Constant4/1 -> alphaBetaLE/2
  Subsystem/2 -> [CD]
  alphaBetaLE/2 -> Terminator/1  "beta_rad"
  [ctrlSurfDefl] -> Subsystem/2
  Subsystem/1 -> [CL]
  Constant6/1 -> Multiply2/4, Multiply3/4
  [vAppLclBdy] -> vAppLclBdy/1
  [dynPress] -> dynPress/1
  [FLiftBdy] -> Add1/1
  [vAppWingTip] -> vAppWingTip/1
  Multiply3/1 -> [FDragBdy], FDragBdy/1
  [dragDirUnitVecBdy] -> Multiply3/3
  [CD] -> CD/1
  [dynPress] -> Multiply2/2
  [alphaLocal] -> Gain/1
  [dynPress] -> Multiply3/2
  [CL] -> CL/1
  [CL] -> Multiply2/1
  [liftDirUnitVecBdy] -> Multiply2/3
  Multiply2/1 -> [FLiftBdy], FLiftBdy/1
  [CD] -> Multiply3/1
  [FDragBdy] -> Add1/2
  Reshape5/1 -> FSumBdy/1
  Cross Product1/1 -> Reshape4/1
  Add1/1 -> Cross Product1/2, Reshape5/1
  Constant7/1 -> Cross Product1/1
  Gain/1 -> alphaLocalDeg/1
  Reshape4/1 -> MBdyAboutLE/1
  Subsystem/3 -> satCtrlSurfDefl/1
  csDeflection/1 -> [ctrlSurfDefl]
  [vAppSurf] -> alphaBetaLE/1
  localApparentWind/2 -> [vAppWingTip]
  [vAppLclBdy] -> DynamicPressure/1
  [vAppLclBdy] -> "  "/2
  DynamicPressure/1 -> [dynPress]
  velBdyWind/1 -> localApparentWind/1
  localApparentWind/1 -> [vAppLclBdy]
  "  "/1 -> [vAppSurf]  "AoAEff"
  alphaBetaLE/1 -> Subsystem/1, [alphaLocal]  "alpha_rad"

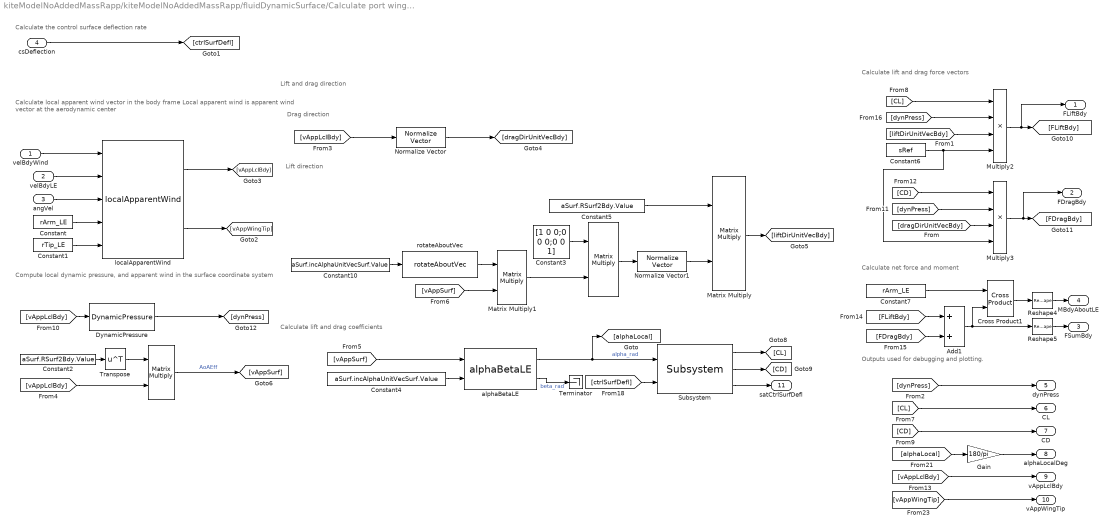
== system kiteModelNoAddedMassRapp/kiteModelNoAddedMassRapp/fluidDynamicSurface/Calculate port wing fluid dynamic loads ==
  note: Calculate the control surface deflection rate
  note: Lift and drag direction
  note: Lift direction
  note: Drag direction
  note: Compute local dynamic pressure,
      | and apparent wind in the surface coordinate system
  note: Calculate local apparent wind vector in the body frame
      | Local apparent wind is apparent wind vector at the aerodynamic center
  note: Calculate lift and drag coefficients
  note: Calculate net force and moment
  note: Outputs used for debugging and plotting.
  note: Calculate lift and drag force vectors
  velBdyWind : Inport
  velBdyLE : Inport  Port=2
  angVel : Inport  Port=3
  csDeflection : Inport  Port=4
  " " : Product  Multiplication=Matrix(*)
  "  " : Product  Multiplication=Matrix(*)
  Add1 : Sum
  Constant : Constant  Value=rArm_LE  VectorParams1D=off
  Constant1 : Constant  Value=rTip_LE  VectorParams1D=off
  Constant10 : Constant  Value=aSurf.incAlphaUnitVecSurf.Value  VectorParams1D=off
  Constant2 : Constant  Value=aSurf.RSurf2Bdy.Value  VectorParams1D=off
  Constant3 : Constant  Value=[1 0 0;0 0 0;0 0 1]  VectorParams1D=off
  Constant4 : Constant  Value=aSurf.incAlphaUnitVecSurf.Value  VectorParams1D=off
  Constant5 : Constant  Value=aSurf.RSurf2Bdy.Value  VectorParams1D=off
  Constant6 : Constant  Value=sRef
  Constant7 : Constant  Value=rArm_LE  VectorParams1D=off
  Cross Product1 : vrlib/Utilities/Cross Product
  DynamicPressure : dynamicPressure_ul/DynamicPressure  rho=fluidDensity
  Gain : Gain  Gain=180/pi
  Matrix Multiply : Product  Multiplication=Matrix(*)
  Matrix Multiply1 : Product  Multiplication=Matrix(*)
  Multiply2 : Product  Inputs=4
  Multiply3 : Product  Inputs=4
  Normalize Vector : vrlib/Utilities/Normalize Vector  maxzero=0
  Normalize Vector1 : vrlib/Utilities/Normalize Vector  maxzero=0
  Reshape4 : Reshape  OutputDimensionality=Column vector (2-D)
  Reshape5 : Reshape  OutputDimensionality=Column vector (2-D)
  Subsystem : Copy_of_clAndCdCalculator_cl/Subsystem  aSurf=aSurf
  Terminator : Terminator
  Transpose : Math  Operator=transpose  SignedPower=on
  alphaBetaLE : alphaBetaLE_ul/alphaBetaLE  SystemSampleTime=-1  VariantActivationTime=update diagram  Latency=0  AutoFrameSizeCalculation=off
  localApparentWind : localApparentWind_ul/localApparentWind  SystemSampleTime=-1  VariantActivationTime=update diagram  Latency=0  AutoFrameSizeCalculation=off
  rotateAboutVec : rotateAboutVec/rotateAboutVec  ang=90
  FLiftBdy : Outport  VectorParamsAs1DForOutWhenUnconnected=off
  FDragBdy : Outport  Port=2  VectorParamsAs1DForOutWhenUnconnected=off
  FSumBdy : Outport  Port=3  VectorParamsAs1DForOutWhenUnconnected=off
  MBdyAboutLE : Outport  Port=4  PortDimensions=[3 1]  VectorParamsAs1DForOutWhenUnconnected=off
  dynPress : Outport  Port=5  VectorParamsAs1DForOutWhenUnconnected=off
  CL : Outport  Port=6  VectorParamsAs1DForOutWhenUnconnected=off
  CD : Outport  Port=7  VectorParamsAs1DForOutWhenUnconnected=off
  alphaLocalDeg : Outport  Port=8  VectorParamsAs1DForOutWhenUnconnected=off
  vAppLclBdy : Outport  Port=9  VectorParamsAs1DForOutWhenUnconnected=off
  vAppWingTip : Outport  Port=10  VectorParamsAs1DForOutWhenUnconnected=off
  satCtrlSurfDefl : Outport  Port=11
  wires:
  velBdyLE/1 -> localApparentWind/2
  angVel/1 -> localApparentWind/3
  Constant/1 -> localApparentWind/4
  Constant1/1 -> localApparentWind/5
  Constant2/1 -> Transpose/1
  Transpose/1 -> "  "/1
  Constant3/1 -> " "/1
  rotateAboutVec/1 -> Matrix Multiply1/1
  Matrix Multiply/1 -> [liftDirUnitVecBdy]
  Normalize Vector1/1 -> Matrix Multiply/2
  Constant10/1 -> rotateAboutVec/1
  Matrix Multiply1/1 -> " "/2
  " "/1 -> Normalize Vector1/1
  Constant5/1 -> Matrix Multiply/1
  [vAppSurf] -> Matrix Multiply1/2
  Normalize Vector/1 -> [dragDirUnitVecBdy]
  [vAppLclBdy] -> Normalize Vector/1
  Constant4/1 -> alphaBetaLE/2
  Subsystem/2 -> [CD]
  alphaBetaLE/2 -> Terminator/1  "beta_rad"
  [ctrlSurfDefl] -> Subsystem/2
  Subsystem/1 -> [CL]
  Constant6/1 -> Multiply2/4, Multiply3/4
  [vAppLclBdy] -> vAppLclBdy/1
  [dynPress] -> dynPress/1
  [FLiftBdy] -> Add1/1
  [vAppWingTip] -> vAppWingTip/1
  Multiply3/1 -> [FDragBdy], FDragBdy/1
  [dragDirUnitVecBdy] -> Multiply3/3
  [CD] -> CD/1
  [dynPress] -> Multiply2/2
  [alphaLocal] -> Gain/1
  [dynPress] -> Multiply3/2
  [CL] -> CL/1
  [CL] -> Multiply2/1
  [liftDirUnitVecBdy] -> Multiply2/3
  Multiply2/1 -> [FLiftBdy], FLiftBdy/1
  [CD] -> Multiply3/1
  [FDragBdy] -> Add1/2
  Reshape5/1 -> FSumBdy/1
  Cross Product1/1 -> Reshape4/1
  Add1/1 -> Cross Product1/2, Reshape5/1
  Constant7/1 -> Cross Product1/1
  Gain/1 -> alphaLocalDeg/1
  Reshape4/1 -> MBdyAboutLE/1
  Subsystem/3 -> satCtrlSurfDefl/1
  csDeflection/1 -> [ctrlSurfDefl]
  [vAppSurf] -> alphaBetaLE/1
  localApparentWind/2 -> [vAppWingTip]
  [vAppLclBdy] -> DynamicPressure/1
  [vAppLclBdy] -> "  "/2
  DynamicPressure/1 -> [dynPress]
  velBdyWind/1 -> localApparentWind/1
  localApparentWind/1 -> [vAppLclBdy]
  "  "/1 -> [vAppSurf]  "AoAEff"
  alphaBetaLE/1 -> Subsystem/1, [alphaLocal]  "alpha_rad"

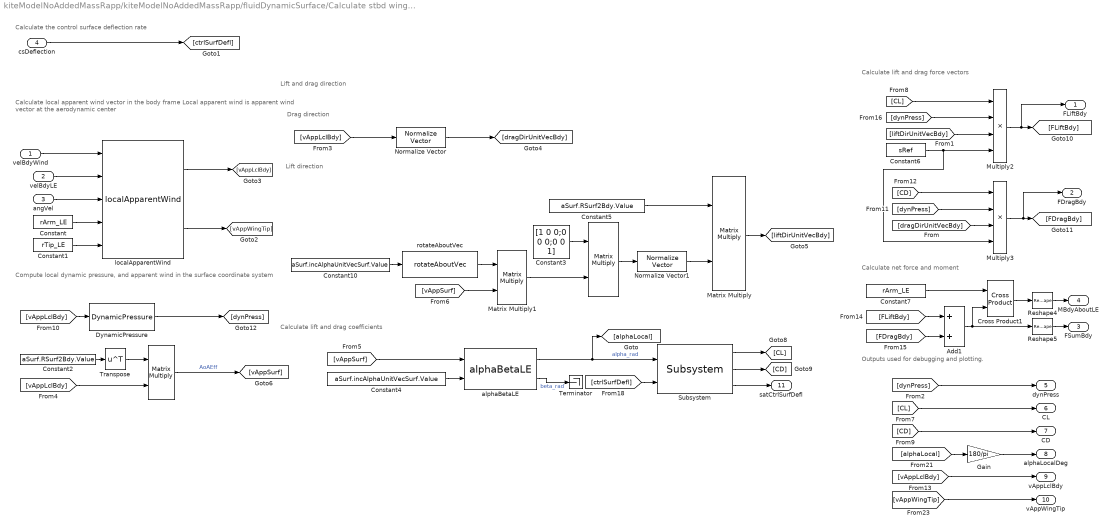
== system kiteModelNoAddedMassRapp/kiteModelNoAddedMassRapp/fluidDynamicSurface/Calculate stbd wing fluid dynamic loads ==
  note: Calculate the control surface deflection rate
  note: Lift and drag direction
  note: Lift direction
  note: Drag direction
  note: Compute local dynamic pressure,
      | and apparent wind in the surface coordinate system
  note: Calculate local apparent wind vector in the body frame
      | Local apparent wind is apparent wind vector at the aerodynamic center
  note: Calculate lift and drag coefficients
  note: Calculate net force and moment
  note: Outputs used for debugging and plotting.
  note: Calculate lift and drag force vectors
  velBdyWind : Inport
  velBdyLE : Inport  Port=2
  angVel : Inport  Port=3
  csDeflection : Inport  Port=4
  " " : Product  Multiplication=Matrix(*)
  "  " : Product  Multiplication=Matrix(*)
  Add1 : Sum
  Constant : Constant  Value=rArm_LE  VectorParams1D=off
  Constant1 : Constant  Value=rTip_LE  VectorParams1D=off
  Constant10 : Constant  Value=aSurf.incAlphaUnitVecSurf.Value  VectorParams1D=off
  Constant2 : Constant  Value=aSurf.RSurf2Bdy.Value  VectorParams1D=off
  Constant3 : Constant  Value=[1 0 0;0 0 0;0 0 1]  VectorParams1D=off
  Constant4 : Constant  Value=aSurf.incAlphaUnitVecSurf.Value  VectorParams1D=off
  Constant5 : Constant  Value=aSurf.RSurf2Bdy.Value  VectorParams1D=off
  Constant6 : Constant  Value=sRef
  Constant7 : Constant  Value=rArm_LE  VectorParams1D=off
  Cross Product1 : vrlib/Utilities/Cross Product
  DynamicPressure : dynamicPressure_ul/DynamicPressure  rho=fluidDensity
  Gain : Gain  Gain=180/pi
  Matrix Multiply : Product  Multiplication=Matrix(*)
  Matrix Multiply1 : Product  Multiplication=Matrix(*)
  Multiply2 : Product  Inputs=4
  Multiply3 : Product  Inputs=4
  Normalize Vector : vrlib/Utilities/Normalize Vector  maxzero=0
  Normalize Vector1 : vrlib/Utilities/Normalize Vector  maxzero=0
  Reshape4 : Reshape  OutputDimensionality=Column vector (2-D)
  Reshape5 : Reshape  OutputDimensionality=Column vector (2-D)
  Subsystem : Copy_of_clAndCdCalculator_cl/Subsystem  aSurf=aSurf
  Terminator : Terminator
  Transpose : Math  Operator=transpose  SignedPower=on
  alphaBetaLE : alphaBetaLE_ul/alphaBetaLE  SystemSampleTime=-1  VariantActivationTime=update diagram  Latency=0  AutoFrameSizeCalculation=off
  localApparentWind : localApparentWind_ul/localApparentWind  SystemSampleTime=-1  VariantActivationTime=update diagram  Latency=0  AutoFrameSizeCalculation=off
  rotateAboutVec : rotateAboutVec/rotateAboutVec  ang=90
  FLiftBdy : Outport  VectorParamsAs1DForOutWhenUnconnected=off
  FDragBdy : Outport  Port=2  VectorParamsAs1DForOutWhenUnconnected=off
  FSumBdy : Outport  Port=3  VectorParamsAs1DForOutWhenUnconnected=off
  MBdyAboutLE : Outport  Port=4  PortDimensions=[3 1]  VectorParamsAs1DForOutWhenUnconnected=off
  dynPress : Outport  Port=5  VectorParamsAs1DForOutWhenUnconnected=off
  CL : Outport  Port=6  VectorParamsAs1DForOutWhenUnconnected=off
  CD : Outport  Port=7  VectorParamsAs1DForOutWhenUnconnected=off
  alphaLocalDeg : Outport  Port=8  VectorParamsAs1DForOutWhenUnconnected=off
  vAppLclBdy : Outport  Port=9  VectorParamsAs1DForOutWhenUnconnected=off
  vAppWingTip : Outport  Port=10  VectorParamsAs1DForOutWhenUnconnected=off
  satCtrlSurfDefl : Outport  Port=11
  wires:
  velBdyLE/1 -> localApparentWind/2
  angVel/1 -> localApparentWind/3
  Constant/1 -> localApparentWind/4
  Constant1/1 -> localApparentWind/5
  Constant2/1 -> Transpose/1
  Transpose/1 -> "  "/1
  Constant3/1 -> " "/1
  rotateAboutVec/1 -> Matrix Multiply1/1
  Matrix Multiply/1 -> [liftDirUnitVecBdy]
  Normalize Vector1/1 -> Matrix Multiply/2
  Constant10/1 -> rotateAboutVec/1
  Matrix Multiply1/1 -> " "/2
  " "/1 -> Normalize Vector1/1
  Constant5/1 -> Matrix Multiply/1
  [vAppSurf] -> Matrix Multiply1/2
  Normalize Vector/1 -> [dragDirUnitVecBdy]
  [vAppLclBdy] -> Normalize Vector/1
  Constant4/1 -> alphaBetaLE/2
  Subsystem/2 -> [CD]
  alphaBetaLE/2 -> Terminator/1  "beta_rad"
  [ctrlSurfDefl] -> Subsystem/2
  Subsystem/1 -> [CL]
  Constant6/1 -> Multiply2/4, Multiply3/4
  [vAppLclBdy] -> vAppLclBdy/1
  [dynPress] -> dynPress/1
  [FLiftBdy] -> Add1/1
  [vAppWingTip] -> vAppWingTip/1
  Multiply3/1 -> [FDragBdy], FDragBdy/1
  [dragDirUnitVecBdy] -> Multiply3/3
  [CD] -> CD/1
  [dynPress] -> Multiply2/2
  [alphaLocal] -> Gain/1
  [dynPress] -> Multiply3/2
  [CL] -> CL/1
  [CL] -> Multiply2/1
  [liftDirUnitVecBdy] -> Multiply2/3
  Multiply2/1 -> [FLiftBdy], FLiftBdy/1
  [CD] -> Multiply3/1
  [FDragBdy] -> Add1/2
  Reshape5/1 -> FSumBdy/1
  Cross Product1/1 -> Reshape4/1
  Add1/1 -> Cross Product1/2, Reshape5/1
  Constant7/1 -> Cross Product1/1
  Gain/1 -> alphaLocalDeg/1
  Reshape4/1 -> MBdyAboutLE/1
  Subsystem/3 -> satCtrlSurfDefl/1
  csDeflection/1 -> [ctrlSurfDefl]
  [vAppSurf] -> alphaBetaLE/1
  localApparentWind/2 -> [vAppWingTip]
  [vAppLclBdy] -> DynamicPressure/1
  [vAppLclBdy] -> "  "/2
  DynamicPressure/1 -> [dynPress]
  velBdyWind/1 -> localApparentWind/1
  localApparentWind/1 -> [vAppLclBdy]
  "  "/1 -> [vAppSurf]  "AoAEff"
  alphaBetaLE/1 -> Subsystem/1, [alphaLocal]  "alpha_rad"

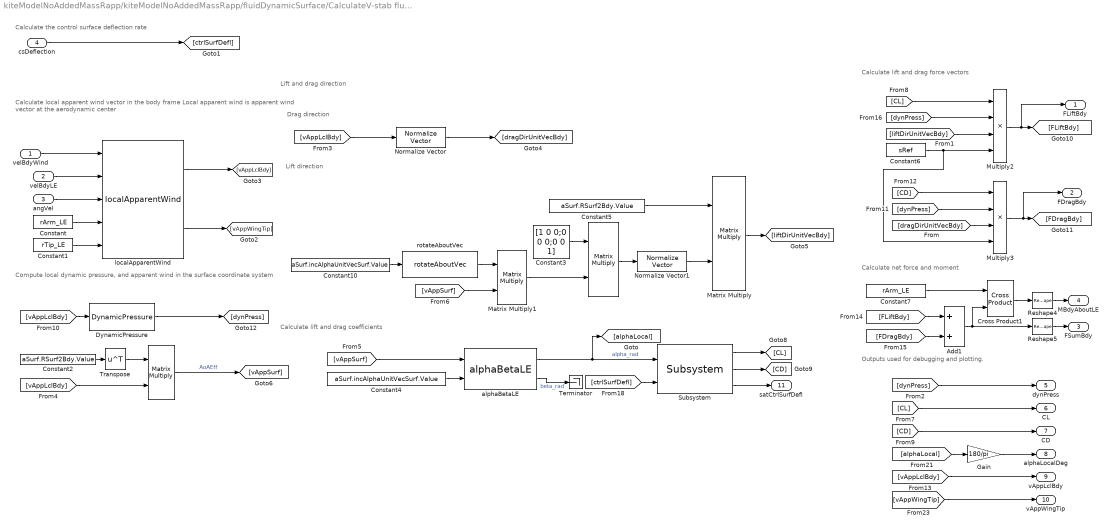
== system kiteModelNoAddedMassRapp/kiteModelNoAddedMassRapp/fluidDynamicSurface/CalculateV-stab fluid dynamic loads ==
  note: Calculate the control surface deflection rate
  note: Lift and drag direction
  note: Lift direction
  note: Drag direction
  note: Compute local dynamic pressure,
      | and apparent wind in the surface coordinate system
  note: Calculate local apparent wind vector in the body frame
      | Local apparent wind is apparent wind vector at the aerodynamic center
  note: Calculate lift and drag coefficients
  note: Calculate net force and moment
  note: Outputs used for debugging and plotting.
  note: Calculate lift and drag force vectors
  velBdyWind : Inport
  velBdyLE : Inport  Port=2
  angVel : Inport  Port=3
  csDeflection : Inport  Port=4
  " " : Product  Multiplication=Matrix(*)
  "  " : Product  Multiplication=Matrix(*)
  Add1 : Sum
  Constant : Constant  Value=rArm_LE  VectorParams1D=off
  Constant1 : Constant  Value=rTip_LE  VectorParams1D=off
  Constant10 : Constant  Value=aSurf.incAlphaUnitVecSurf.Value  VectorParams1D=off
  Constant2 : Constant  Value=aSurf.RSurf2Bdy.Value  VectorParams1D=off
  Constant3 : Constant  Value=[1 0 0;0 0 0;0 0 1]  VectorParams1D=off
  Constant4 : Constant  Value=aSurf.incAlphaUnitVecSurf.Value  VectorParams1D=off
  Constant5 : Constant  Value=aSurf.RSurf2Bdy.Value  VectorParams1D=off
  Constant6 : Constant  Value=sRef
  Constant7 : Constant  Value=rArm_LE  VectorParams1D=off
  Cross Product1 : vrlib/Utilities/Cross Product
  DynamicPressure : dynamicPressure_ul/DynamicPressure  rho=fluidDensity
  Gain : Gain  Gain=180/pi
  Matrix Multiply : Product  Multiplication=Matrix(*)
  Matrix Multiply1 : Product  Multiplication=Matrix(*)
  Multiply2 : Product  Inputs=4
  Multiply3 : Product  Inputs=4
  Normalize Vector : vrlib/Utilities/Normalize Vector  maxzero=0
  Normalize Vector1 : vrlib/Utilities/Normalize Vector  maxzero=0
  Reshape4 : Reshape  OutputDimensionality=Column vector (2-D)
  Reshape5 : Reshape  OutputDimensionality=Column vector (2-D)
  Subsystem : Copy_of_clAndCdCalculator_cl/Subsystem  aSurf=aSurf
  Terminator : Terminator
  Transpose : Math  Operator=transpose  SignedPower=on
  alphaBetaLE : alphaBetaLE_ul/alphaBetaLE  SystemSampleTime=-1  VariantActivationTime=update diagram  Latency=0  AutoFrameSizeCalculation=off
  localApparentWind : localApparentWind_ul/localApparentWind  SystemSampleTime=-1  VariantActivationTime=update diagram  Latency=0  AutoFrameSizeCalculation=off
  rotateAboutVec : rotateAboutVec/rotateAboutVec  ang=90
  FLiftBdy : Outport  VectorParamsAs1DForOutWhenUnconnected=off
  FDragBdy : Outport  Port=2  VectorParamsAs1DForOutWhenUnconnected=off
  FSumBdy : Outport  Port=3  VectorParamsAs1DForOutWhenUnconnected=off
  MBdyAboutLE : Outport  Port=4  PortDimensions=[3 1]  VectorParamsAs1DForOutWhenUnconnected=off
  dynPress : Outport  Port=5  VectorParamsAs1DForOutWhenUnconnected=off
  CL : Outport  Port=6  VectorParamsAs1DForOutWhenUnconnected=off
  CD : Outport  Port=7  VectorParamsAs1DForOutWhenUnconnected=off
  alphaLocalDeg : Outport  Port=8  VectorParamsAs1DForOutWhenUnconnected=off
  vAppLclBdy : Outport  Port=9  VectorParamsAs1DForOutWhenUnconnected=off
  vAppWingTip : Outport  Port=10  VectorParamsAs1DForOutWhenUnconnected=off
  satCtrlSurfDefl : Outport  Port=11
  wires:
  velBdyLE/1 -> localApparentWind/2
  angVel/1 -> localApparentWind/3
  Constant/1 -> localApparentWind/4
  Constant1/1 -> localApparentWind/5
  Constant2/1 -> Transpose/1
  Transpose/1 -> "  "/1
  Constant3/1 -> " "/1
  rotateAboutVec/1 -> Matrix Multiply1/1
  Matrix Multiply/1 -> [liftDirUnitVecBdy]
  Normalize Vector1/1 -> Matrix Multiply/2
  Constant10/1 -> rotateAboutVec/1
  Matrix Multiply1/1 -> " "/2
  " "/1 -> Normalize Vector1/1
  Constant5/1 -> Matrix Multiply/1
  [vAppSurf] -> Matrix Multiply1/2
  Normalize Vector/1 -> [dragDirUnitVecBdy]
  [vAppLclBdy] -> Normalize Vector/1
  Constant4/1 -> alphaBetaLE/2
  Subsystem/2 -> [CD]
  alphaBetaLE/2 -> Terminator/1  "beta_rad"
  [ctrlSurfDefl] -> Subsystem/2
  Subsystem/1 -> [CL]
  Constant6/1 -> Multiply2/4, Multiply3/4
  [vAppLclBdy] -> vAppLclBdy/1
  [dynPress] -> dynPress/1
  [FLiftBdy] -> Add1/1
  [vAppWingTip] -> vAppWingTip/1
  Multiply3/1 -> [FDragBdy], FDragBdy/1
  [dragDirUnitVecBdy] -> Multiply3/3
  [CD] -> CD/1
  [dynPress] -> Multiply2/2
  [alphaLocal] -> Gain/1
  [dynPress] -> Multiply3/2
  [CL] -> CL/1
  [CL] -> Multiply2/1
  [liftDirUnitVecBdy] -> Multiply2/3
  Multiply2/1 -> [FLiftBdy], FLiftBdy/1
  [CD] -> Multiply3/1
  [FDragBdy] -> Add1/2
  Reshape5/1 -> FSumBdy/1
  Cross Product1/1 -> Reshape4/1
  Add1/1 -> Cross Product1/2, Reshape5/1
  Constant7/1 -> Cross Product1/1
  Gain/1 -> alphaLocalDeg/1
  Reshape4/1 -> MBdyAboutLE/1
  Subsystem/3 -> satCtrlSurfDefl/1
  csDeflection/1 -> [ctrlSurfDefl]
  [vAppSurf] -> alphaBetaLE/1
  localApparentWind/2 -> [vAppWingTip]
  [vAppLclBdy] -> DynamicPressure/1
  [vAppLclBdy] -> "  "/2
  DynamicPressure/1 -> [dynPress]
  velBdyWind/1 -> localApparentWind/1
  localApparentWind/1 -> [vAppLclBdy]
  "  "/1 -> [vAppSurf]  "AoAEff"
  alphaBetaLE/1 -> Subsystem/1, [alphaLocal]  "alpha_rad"

== matlab function kiteModelNoAddedMassRapp/MATLAB Function ==
  data: a_a input; body2Aero output; b_a input
function body2Aero = fcn(a_a,b_a)
a = a_a; 
b = b_a;

body2Aero = [cos(a)*cos(b), sin(b), sin(a)*cos(b);
             -cos(a)*sin(b), cos(b), -sin(a)*sin(b);
             -sin(a) 0 cos(a)];

== matlab function kiteModelNoAddedMassRapp/MATLAB Function2 ==
  data: az input; wind2Tangent output; el input
function wind2Tangent = fcn(az,el)

wind2Tangent = [-sin(el)*cos(az),-sin(el)*sin(az),cos(el);
    -sin(az), cos(az), 0 ; 
    -cos(el)*cos(az),-cos(el)*sin(az), -sin(el)];

== matlab function kiteModelNoAddedMassRapp/states 4-6/MATLAB Function ==
  data: phi_t input; matMult output; theta_t input; psi_t input
function matMult = fcn(phi_t,theta_t,psi_t)

matMult= [1,sin(psi_t)*tan(theta_t),cos(phi_t)*tan(theta_t);
    0, cos(phi_t),-sin(phi_t);
    0, sin(phi_t)/cos(theta_t), cos(phi_t)/cos(theta_t)];

== matlab function kiteModelNoAddedMassRapp/MATLAB Function1 ==
  data: phiT input; body2Tangent output; thetaT input; psiT input
function body2Tangent = fcn(phiT,thetaT,psiT)

body2Tangent = [cos(psiT)*cos(thetaT),cos(psiT)*sin(phiT)*sin(thetaT)-cos(phiT)*sin(psiT), sin(phiT)*sin(psiT)+cos(phiT)*cos(psiT)*sin(thetaT);
    cos(thetaT)*sin(psiT), cos(phiT)*cos(psiT)+sin(phiT)*sin(psiT)*sin(thetaT),cos(phiT)*sin(psiT)*sin(thetaT)-cos(psiT)*sin(phiT)
    -sin(thetaT), cos(thetaT)*sin(phiT),cos(phiT)*cos(thetaT)];
